simulink model "HybridSimulator"  (Simulink 7.8)
settings: Solver=ode45  StartTime=0.0  StopTime=T  MaxStep=MaxStep  RelTol=RelTol
model workspace (MAT data in the model file):
  statevect : Simulink.Signal (value not decoded)
  inputvect : Simulink.Signal (value not decoded)
  M : Simulink.Signal (value not decoded)
  CLmax : Simulink.Signal (value not decoded)
  CD0 : Simulink.Signal (value not decoded)
  K : Simulink.Signal (value not decoded)
  Sref : Simulink.Signal (value not decoded)
  Tmax : Simulink.Signal (value not decoded)
  G : Simulink.Signal (value not decoded)
  Rho : Simulink.Signal (value not decoded)
  Rc : Simulink.Signal (value not decoded)
  mu : Simulink.Signal (value not decoded)
  p : Simulink.Signal (value not decoded)
  Vc1 : Simulink.Signal (value not decoded)
  Vc2 : Simulink.Signal (value not decoded)
  d : Simulink.Signal (value not decoded)
  c : Simulink.Signal (value not decoded)
  Tmin : Simulink.Signal (value not decoded)
values from neighbouring files (symbols this model uses):
  J = 5    [initialization.m]    (also in plotHybridArc.m = j(length(j)); plotflows.m = j(length(j)); plotjumps.m = j(length(j)))
  rule = 1    [initialization.m]
  T = 120    [initialization.m]    (also in plotHybridArc.m = t(length(t)); plotflows.m = t(length(t)); plotjumps.m = t(length(t)))
  x0 = [X0; Y0; V0; Psi0; q0]    [initialization.m]
  z0 = [x0; u0]    [initialization.m]
libraries: simulink x2
CloseFcn:
  | rtwprivate ssgencode ModelCloseRequest HybridSimulator
settings Model: Creator=rsanfelice  LastModifiedBy=Dean3  ExtModeAutoUpdateStatusClock=off
settings SolverCC: ZeroCrossControl=DisableAll
settings DataIOCC: LimitDataPoints=off  SaveOutput=off  SignalLogging=off  DSMLogging=off  SaveTime=off
settings OptimizationCC: EnhancedBackFolding=on  InitFltsAndDblsToZero=on  SimCompilerOptimization=On
settings DebuggingCC: AlgebraicLoopMsg=none  SaveWithParameterizedLinksMsg=none  SignalResolutionControl=TryResolveAllWithWarning  SolverPrmCheckMsg=none  MultiTaskDSMMsg=warning  MultiTaskCondExecSysMsg=none  FcnCallInpInsideContextMsg=Use local settings  StrictBusMsg=None
settings HardwareCC: TargetIntDivRoundTo=Zero  TargetEndianess=LittleEndian  TargetHWDeviceType=MATLAB Host  ProdEqTarget=off
settings RTWCC: IncludeERTFirstTime=on
settings GRTTargetCC: TargetFcnLib=ansi_tfl_tmw.mat

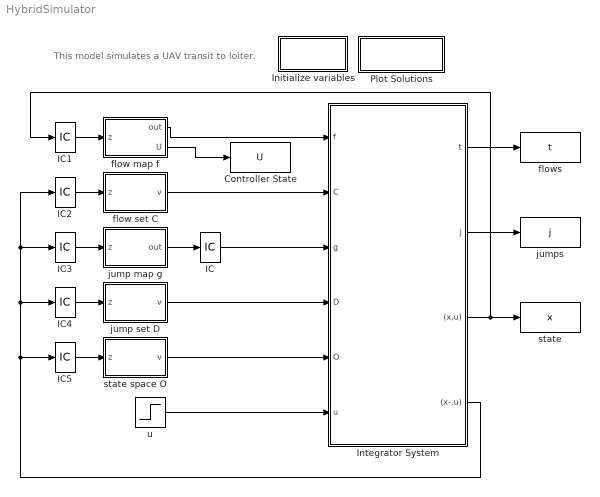
== system HybridSimulator ==
  note: This model simulates a UAV transit to loiter.
  Controller State : ToWorkspace  VariableName=U  SampleTime=-1  SaveFormat=Array
  IC : InitialCondition  Value=x0
  IC{1..5} (5 alike) : InitialCondition  Value=z0
  Initialize variables : Subsystem
      settings: OpenFcn=initialization
      mask Display: disp('Double Click\n to Initialize')
  Integrator System : Subsystem
  Plot Solutions : Subsystem
      settings: OpenFcn=postprocessing
      mask Display: disp('Double Click to\n Plot Solutions')
  flow map f : MATLAB Function  TreatAsAtomicUnit=on
  flow set C : MATLAB Function  TreatAsAtomicUnit=on
  flows : ToWorkspace  VariableName=t  SampleTime=-1  SaveFormat=Array
  jump map g : MATLAB Function  TreatAsAtomicUnit=on
  jump set D : MATLAB Function  TreatAsAtomicUnit=on
  jumps : ToWorkspace  VariableName=j  SampleTime=-1  SaveFormat=Array
  state : ToWorkspace  VariableName=x  SampleTime=-1  SaveFormat=Array
  state space O : MATLAB Function  TreatAsAtomicUnit=on
  u : Step  Time=0  After=0  SampleTime=0
  wires:
  flow map f/1(out) -> Integrator System/1(f)
  Integrator System/4("(x-,u) ") -> IC5/1, IC4/1, IC3/1, IC2/1
  Integrator System/3((x,u)) -> state/1, IC1/1
  flow set C/1(v) -> Integrator System/2(C)
  Integrator System/1(t) -> flows/1
  Integrator System/2(j) -> jumps/1
  state space O/1(v) -> Integrator System/5(O)
  u/1 -> Integrator System/6(u)
  IC1/1 -> flow map f/1(z)
  IC5/1 -> state space O/1(z)
  IC3/1 -> jump map g/1(z)
  jump set D/1(v) -> Integrator System/4(D)
  jump map g/1(out) -> IC/1
  IC/1 -> Integrator System/3(g)
  flow map f/2(U) -> Controller State/1
  IC2/1 -> flow set C/1(z)
  IC4/1 -> jump set D/1(z)

== system HybridSimulator/Initialize variables ==

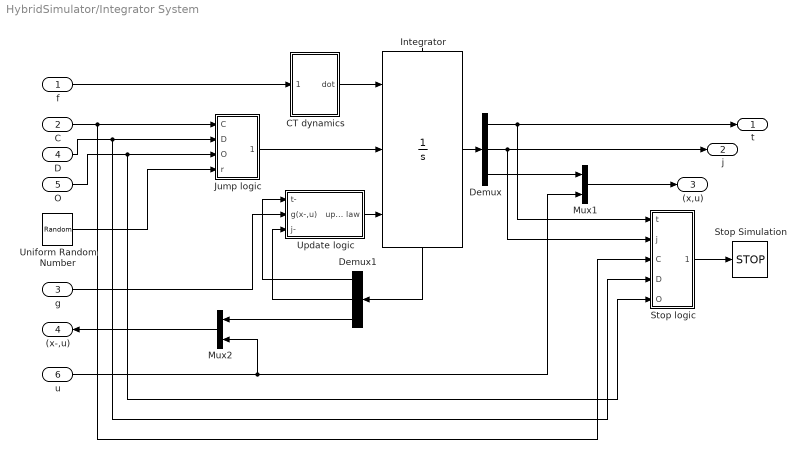
== system HybridSimulator/Integrator System ==
  f : Inport
  C : Inport  Port=2
  g : Inport  Port=3
  D : Inport  Port=4
  O : Inport  Port=5
  u : Inport  Port=6
  CT dynamics : Subsystem
  Demux : Demux  Outputs=[1 1 -1]
  Demux1 : Demux  Outputs=[1 1 -1]
  Integrator : Integrator  ExternalReset=level hold  InitialConditionSource=external  ShowStatePort=on  ZeroCross=off
  Jump logic : Subsystem
  Mux1 : Mux  Inputs=2
  Mux2 : Mux  Inputs=2
  Stop Simulation : Stop
  Stop logic : Subsystem
  Uniform Random Number : UniformRandomNumber  Minimum=0  Seed=abs(floor(100*rand))  SampleTime=0
  Update logic : Subsystem
  t : Outport
  j : Outport  Port=2
  (x,u) : Outport  Port=3
  "(x-,u) " : Outport  Port=4
  wires:
  Demux/2 -> j/1, Stop logic/2(j)
  Demux/1 -> t/1, Stop logic/1(t)
  Demux1/2 -> Update logic/3(j-)
  Demux1/1 -> Update logic/1(t-)
  Update logic/1(update law) -> Integrator/3
  Integrator/State -> Demux1/1
  CT dynamics/1(dot) -> Integrator/1
  Stop logic/1(stop) -> Stop Simulation/1
  Integrator/1 -> Demux/1
  C/1 -> Jump logic/1(C), Stop logic/3(C)
  D/1 -> Jump logic/2(D), Stop logic/4(D)
  O/1 -> Jump logic/3(O), Stop logic/5(O)
  f/1 -> CT dynamics/1(f(x,u))
  Demux1/3 -> Mux2/1
  g/1 -> Update logic/2(g(x-,u))
  Jump logic/1(jump) -> Integrator/2
  Uniform Random Number/1 -> Jump logic/4(r)
  Demux/3 -> Mux1/1
  Mux1/1 -> (x,u)/1
  u/1 -> Mux2/2, Mux1/2
  Mux2/1 -> "(x-,u) "/1

== system HybridSimulator/Plot Solutions ==

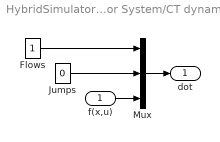
== system HybridSimulator/Integrator System/CT dynamics ==
  f(x,u) : Inport
  Flows : Constant
  Jumps : Constant  Value=0
  Mux : Mux  Inputs=[1 1 -1]
  dot : Outport
  wires:
  Jumps/1 -> Mux/2
  Flows/1 -> Mux/1
  Mux/1 -> dot/1
  f(x,u)/1 -> Mux/3

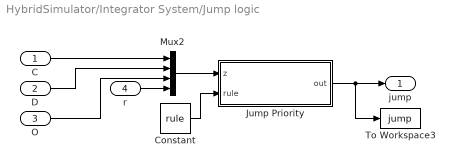
== system HybridSimulator/Integrator System/Jump logic ==
  C : Inport
  D : Inport  Port=2
  O : Inport  Port=3
  r : Inport  Port=4
  Constant : Constant  Value=rule
  Jump Priority : MATLAB Function  TreatAsAtomicUnit=on
  Mux2 : Mux
  To Workspace3 : ToWorkspace  VariableName=jump  SampleTime=-1  SaveFormat=Array
  jump : Outport
  wires:
  Mux2/1 -> Jump Priority/1(z)
  Jump Priority/1(out) -> jump/1, To Workspace3/1
  C/1 -> Mux2/1
  r/1 -> Mux2/4
  D/1 -> Mux2/2
  O/1 -> Mux2/3
  Constant/1 -> Jump Priority/2(rule)

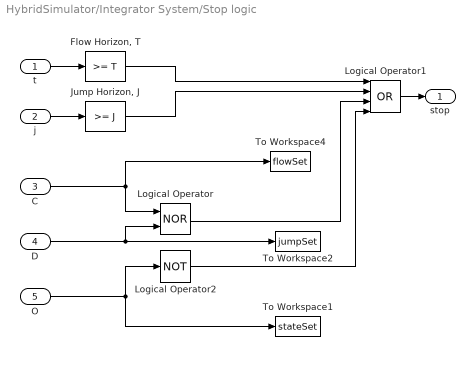
== system HybridSimulator/Integrator System/Stop logic ==
  t : Inport
  j : Inport  Port=2
  C : Inport  Port=3
  D : Inport  Port=4
  O : Inport  Port=5
  "Flow Horizon, T" : simulink/Logic and Bit Operations/Compare To Constant  relop=>=  const=T  OutDataTypeStr=uint8  ZeroCross=off
  "Jump Horizon, J" : simulink/Logic and Bit Operations/Compare To Constant  relop=>=  const=J  OutDataTypeStr=uint8  ZeroCross=off
  Logical Operator : Logic  Operator=NOR  AllPortsSameDT=off  OutDataTypeStr=boolean
  Logical Operator1 : Logic  Operator=OR  Inputs=4  AllPortsSameDT=off  OutDataTypeStr=boolean
  Logical Operator2 : Logic  Operator=NOT  AllPortsSameDT=off  OutDataTypeStr=boolean
  To Workspace1 : ToWorkspace  VariableName=stateSet  SampleTime=-1  SaveFormat=Array
  To Workspace2 : ToWorkspace  VariableName=jumpSet  SampleTime=-1  SaveFormat=Array
  To Workspace4 : ToWorkspace  VariableName=flowSet  SampleTime=-1  SaveFormat=Array
  stop : Outport
  wires:
  "Flow Horizon, T"/1 -> Logical Operator1/1
  "Jump Horizon, J"/1 -> Logical Operator1/2
  Logical Operator/1 -> Logical Operator1/3
  Logical Operator2/1 -> Logical Operator1/4
  D/1 -> Logical Operator/2, To Workspace2/1
  O/1 -> Logical Operator2/1, To Workspace1/1
  t/1 -> "Flow Horizon, T"/1
  j/1 -> "Jump Horizon, J"/1
  C/1 -> Logical Operator/1, To Workspace4/1
  Logical Operator1/1 -> stop/1

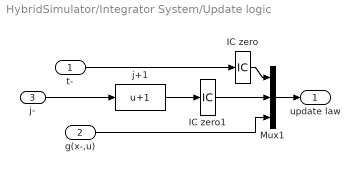
== system HybridSimulator/Integrator System/Update logic ==
  t- : Inport
  g(x-,u) : Inport  Port=2
  j- : Inport  Port=3
  IC zero : InitialCondition  Value=0
  IC zero1 : InitialCondition  Value=0
  Mux1 : Mux  Inputs=[1 1 -1]
  j+1 : MATLABFcn  MATLABFcn=u+1
  update law : Outport
  wires:
  IC zero1/1 -> Mux1/2
  j+1/1 -> IC zero1/1
  IC zero/1 -> Mux1/1
  t-/1 -> IC zero/1
  Mux1/1 -> update law/1
  j-/1 -> j+1/1
  g(x-,u)/1 -> Mux1/3

== matlab function jump set D ==
  data: v output double; statevect data_store_memory double; inputvect data_store_memory double; M data_store_memory double; CLmax data_store_memory double; CD0 data_store_memory double; K data_store_memory double; Sref data_store_memory double; Tmax data_store_memory double; G data_store_memory double; Rho data_store_memory double; Rc data_store_memory double; Vc1 data_store_memory double; c data_store_memory double; d data_store_memory double; Tmin data_store_memory double; p data_store_memory double; z input double; mu data_store_memory double
function v  = D(z) 
%%%%%%%%%%%%%%%%%%%%%%%%%%%%%%%%%%%%%%%%%%%%%%%%%%%%%%%%%%%%%%%%%%%%%%%%%%%%%%%%%%%%%%%%%%%%%%%%%%
% Matlab M-file                Author: Dean Smith
%
% Project: Simulation of a hybrid system (UAV waypoint loitering)
%
%
% Name: D.m
%
% Description: Jump set
%
% Version: 0.6
% Required files: - 
%%%%%%%%%%%%%%%%%%%%%%%%%%%%%%%%%%%%%%%%%%%%%%%%%%%%%%%%%%%%%%%%%%%%%%%%%%%%%%%%%%%%%%%%%%%%%%%%%%

% constants
global statevect inputvect M CLmax CD0 K Sref Tmax G Rho Rc Vc1 c d Tmin p mu;
    %n = # of state components
    %m = # of input components 

% state
%x = z(1:n);
x = z(statevect);
X = x(1);      
Y = x(2);           
V = x(3);      
Psi = x(4);
q = x(5);    

%input
%u = z(n+1:n+m);
%u = z(inputvect);

%Intermediate Calculation
R = sqrt(X^2 + Y^2);
[Psi_c,junk] = PsiC(X,Y,V,Psi,1,p,Rc,mu);

v=0; %case to get function to compile
switch q 
    case 1 %local
        if abs(R-Rc) >= d % jump condition
            v = 1;  % report jump
        else
            v = 0;   % do not report jump
        end
    case 2; %global
        if 0.5*((R-Rc)^2+(V-Vc1)^2+(Psi-Psi_c)^2) <= c % jump condition
            v = 1;  % report jump
        else
            v = 0;   % do not report jump
        end 
end

== matlab function flow map f ==
  data: mu data_store_memory double; z input double; out output double; statevect data_store_memory double; inputvect data_store_memory double; M data_store_memory double; CLmax data_store_memory double; CD0 data_store_memory double; K data_store_memory double; Sref data_store_memory double; Tmax data_store_memory double; G data_store_memory double; Rho data_store_memory double; Vc1 data_store_memory double; Vc2 data_store_memory double; Rc data_store_memory double; p data_store_memory double; U output double; Tmin data_store_memory double
function [out, U] = f(z)
%%%%%%%%%%%%%%%%%%%%%%%%%%%%%%%%%%%%%%%%%%%%%%%%%%%%%%%%%%%%%%%%%%%%%%%%%%%%%%%%%%%%%%%%%%%%%%%%%%
% Matlab M-file              Author: Dean Smith
%
% Project: Simulation of a hybrid system (UAV waypoint loitering)
%
% Name: f.m
%
% Description: Flow map
%
% Version: 0.6
% Required files: -
%%%%%%%%%%%%%%%%%%%%%%%%%%%%%%%%%%%%%%%%%%%%%%%%%%%%%%%%%%%%%%%%%%%%%%%%%%%%%%%%%%%%%%%%%%%%%%%%%%

% constants
global statevect inputvect M CLmax CD0 K Sref Tmax G Rho Rc Vc1 Vc2 mu p Tmin;
% n = # of state components
% m = # of input components

% state
%x = z(1:n);
x = z(statevect);
X = x(1);
Y = x(2);
V = x(3);
Psi = x(4);
q = x(5);

%input
%u = z(n+1:n+m);
%u = z(inputvect);

%Intermediate Calculation
W = M*G; %weight N
R = sqrt(X^2 + Y^2);
qa = 0.5*Rho*V^2; %current dynamic pressure
PhiMax = acos(W/(Sref*qa*CLmax));

%Controller Gains
k_T1 = 1000;
k_T2 = 1000;

%limit Psi to +/-180
while Psi < -pi
    Psi = Psi + 2*pi;
end
while Psi > pi
    Psi = Psi - 2*pi;
end
Psi = rem(Psi,2*pi);

%Initialize so code will compile
k_Phi = 0;
k_T = 0;
Vc = 0;
Psi_c = Psi;
%Determine Desired Heading
[Psi_c,p] = PsiC(X,Y,V,Psi,q,p,Rc,mu);
Delta = Psi-Psi_c;

%limit Delta to +/-180
while Delta < -pi
    Delta = Delta + 2*pi;
end
while Delta > pi
    Delta = Delta - 2*pi;
end
Delta = rem(Delta,2*pi);

switch q
    case 1 %local
        Chi = 10;
%         if abs(Delta) >= pi/2
%             gamma = 0.75;
%         else
%             gamma = 0;
%         end
        gamma = 3/2/pi*abs(Delta);

       % if sign(R-Rc)*p*sign(sin(Delta)) < 0
%             beta=1-1e-6;
%             zeta = asin(max(0,min(beta*abs(R^2-Rc^2)/(2*R*Rc),1)));
     %   else
     %       zeta = 1;
     %   end
       zeta = 10*pi/180;
      

        k_Phi = Chi+gamma*V*(R-Rc)^2*(Rc+R)/(Rc^2+R^2)+ abs(sin(Delta))/zeta^2*V*2*R*Rc*abs(R-Rc)/(Rc^2+R^2);
    case 2 %global
        nu = 10;
%         if abs(Delta) >= pi/2
%             xsi = 0.75;
%         else
%             xsi = 0;
%         end
        xsi = 3/2/pi*abs(Delta);
        k_Phi = nu+xsi*V*abs(R-Rc);
end

%Calculate Bank Angle (Phi) Control Input
if R == 0
    Phi_C = 0;
else
    Phi_C = atan( -k_Phi*Delta*V/G - Y*V^2/(G*R^2)*cos(Psi) + X*V^2/(G*R^2)*sin(Psi) );
end

%limit Phi to +/-180
while Phi_C < -pi
    Phi_C = Phi_C + 2*pi;
end
while Phi_C > pi
    Phi_C = Phi_C - 2*pi;
end

%make sure bank angle does not exceed limit
if Phi_C > PhiMax
    Phi_C = PhiMax;
elseif Phi_C < -PhiMax
    Phi_C = -PhiMax;
end

%Calculate Drag Force
CL = W/(Sref*qa*cos(Phi_C));

CD = CD0 + K*CL^2;
D = CD*Sref*qa;

%determine thrust command
switch q
    case 1 %local
        Vc = Vc1;
        k_T = k_T1;
    case 2 %global
        Vc = Vc2;
        k_T = k_T2;
end
T = D - k_T*(V-Vc);

%Limit thrust
T = max(min(T,Tmax),Tmin);

% flow map
x1dot = V*cos(Psi);
x2dot = V*sin(Psi);
x3dot = (T-D)/M;
x4dot = G/V*tan(Phi_C);
x5dot = 0;
out = [x1dot;x2dot;x3dot;x4dot;x5dot];
U = [atan(Phi_C); T; Psi_c; D];

== matlab function state space O ==
  data: z input double; v output double; statevect data_store_memory double; inputvect data_store_memory double
function v  = O(z) 
%%%%%%%%%%%%%%%%%%%%%%%%%%%%%%%%%%%%%%%%%%%%%%%%%%%%%%%%%%%%%%%%%%%%%%%%%%%%%%%%%%%%%%%%%%%%%%%%%%
% Matlab M-file                Author: Ricardo Sanfelice
%
% Project: Simulation of a hybrid system (Bouncing ball)
%
%
% Name: O.m
%
% Description: State space
%
% Version: 0.6
% Required files: - 
%%%%%%%%%%%%%%%%%%%%%%%%%%%%%%%%%%%%%%%%%%%%%%%%%%%%%%%%%%%%%%%%%%%%%%%%%%%%%%%%%%%%%%%%%%%%%%%%%%


v = 1;

== matlab function Integrator System/Jump logic/Jump Priority ==
  data: z input double; out output double; statevect data_store_memory double; inputvect data_store_memory double; rule input double
function out = jumpPriority(z,rule)
%%%%%%%%%%%%%%%%%%%%%%%%%%%%%%%%%%%%%%%%%%%%%%%%%%%%%%%%%%%%%%%%%%%%%%%%%%%
% Matlab M-file                Author: Ricardo Sanfelice
%
% Project: Simulation of a hybrid system
%
%
% Name: jumpPriority.m
%
% Description: Jump priority function
%
% Version: 0.6
% Required files: -
%%%%%%%%%%%%%%%%%%%%%%%%%%%%%%%%%%%%%%%%%%%%%%%%%%%%%%%%%%%%%%%%%%%%%%%%%%%

% state
flowFlag = z(1);
jumpFlag = z(2);
stateFlag = z(3);
randomInput = z(4);

% rule = 1 -> priority for jumps
% rule = 2 -> priority for flows
% rule = 3 -> no priority, random selection when simultaneous conditions

if (rule == 1) && (jumpFlag == 1)
   out = 1;
elseif (rule == 1) && (jumpFlag == 0)
   out = 0;
elseif (rule == 2) && (flowFlag == 1)
   out = 0;
elseif (rule == 2) && (flowFlag == 0) && (jumpFlag == 0)
   out = 0;
elseif (rule == 2) && (flowFlag == 0) && (jumpFlag == 1)
   out = 1;
elseif (rule == 3)
   if (flowFlag == 1) && (jumpFlag == 0)
      out = 0;
   elseif (flowFlag == 0) && (jumpFlag == 1)
      out = 1;
   elseif (flowFlag == 1) && (jumpFlag == 1)
%      aux = 0.4 + (0.6-0.4).*rand;
      if (randomInput >= 0.5)
         out = 1;
      else
         out = 0;
      end
   else
       out = 0;
   end
else 
    out = 0;
end

== matlab function flow set C ==
  data: v output double; z input double; statevect data_store_memory double; inputvect data_store_memory double; M data_store_memory double; CLmax data_store_memory double; CD0 data_store_memory double; K data_store_memory double; Sref data_store_memory double; Tmax data_store_memory double; G data_store_memory double; Rho data_store_memory double; Rc data_store_memory double; Vc1 data_store_memory double; d data_store_memory double; c data_store_memory double; Tmin data_store_memory double; p data_store_memory double; mu data_store_memory double
function v  = C(z) 
%%%%%%%%%%%%%%%%%%%%%%%%%%%%%%%%%%%%%%%%%%%%%%%%%%%%%%%%%%%%%%%%%%%%%%%%%%%%%%%%%%%%%%%%%%%%%%%%%%
% Matlab M-file                Author: Dean Smith
%
% Project: Simulation of a hybrid system (UAV waypoint loitering)
%
% Name: C.m
%
% Description: Flow set
%
% Version: 0.6
% Required files: - 
%%%%%%%%%%%%%%%%%%%%%%%%%%%%%%%%%%%%%%%%%%%%%%%%%%%%%%%%%%%%%%%%%%%%%%%%%%%%%%%%%%%%%%%%%%%%%%%%%%

% constants
global statevect inputvect M CLmax CD0 K Sref Tmax G Rho Rc Vc1 d c Tmin p mu;
    %n = # of state components
    %m = # of input components 

% state
%x = z(1:n);
x = z(statevect);
X = x(1);      
Y = x(2);           
V = x(3);      
Psi = x(4);
q = x(5);      

%input
%u = z(n+1:n+m);
%u = z(inputvect);

%Intermediate Calculation
R = sqrt(X^2 + Y^2);
[Psi_c,junk] = PsiC(X,Y,V,Psi,1,p,Rc,mu);

v=0; %case to get function to compile
switch q 
    case 1 %local
        if abs(R-Rc) <= d % flow condition
            v = 1;  % report flow
        else
            v = 0;   % do not report flow
        end
    case 2 %global
        if 0.5*((R-Rc)^2+(V-Vc1)^2+(Psi-Psi_c)^2) >= c % flow condition
            v = 1;  % report flow
        else
            v = 0;   % do not report flow
        end 
end

== matlab function jump map g ==
  data: z input double; out output double; statevect data_store_memory double; inputvect data_store_memory double; M data_store_memory double; CLmax data_store_memory double; CD0 data_store_memory double; K data_store_memory double; Sref data_store_memory double; Tmax data_store_memory double; G data_store_memory double; Rho data_store_memory double; Tmin data_store_memory double
function out = g(z)
%%%%%%%%%%%%%%%%%%%%%%%%%%%%%%%%%%%%%%%%%%%%%%%%%%%%%%%%%%%%%%%%%%%%%%%%%%%
% Matlab M-file                Author: Dean Smith
%
% Project: Simulation of a hybrid system (UAV waypoint loitering)
%
%
% Name: g.m
%
% Description: Jump map
%
% Version: 0.6
% Required files: - 
%%%%%%%%%%%%%%%%%%%%%%%%%%%%%%%%%%%%%%%%%%%%%%%%%%%%%%%%%%%%%%%%%%%%%%%%%%%

% constants
global  statevect inputvect;
    %n = # of state components
    %m = # of input components 

% state
%x = z(1:n);
x = z(statevect);
X = x(1);      
Y = x(2);           
V = x(3);      
Psi = x(4);
q = x(5);     

x1plus = X;
x2plus = Y;
x3plus = V;
x4plus = Psi;
x5plus = 3-q;

out = [x1plus;x2plus;x3plus;x4plus;x5plus];
